simulink model "Ex9"  (R2019b)
settings: Solver=VariableStepAuto  StartTime=0.0  StopTime=0.003  RelTol=1e-3
values from neighbouring files (symbols this model uses):
  C = 1 / (L*Wn^2)    (= 2.29568411387e-06)    [Ex_27.m]    (also in Ex_29.m = 0.0001; Ex_5.m = 1e-06; Ex_8.m = 1e-05; Ex_9.m = 1e-05)
  L = 0.2    [Ex_23.m]    (also in Ex_27.m = 0.0001; Ex_29.m; Ex_8.m = 0.001; Ex_9.m = 0.001)
  R = 0.2    [Ex_21.m]    (also in Ex_22.m; Ex_23.m = 1.3; Ex_27.m = 2*qsi * sqrt(L/C); Ex_29.m = 1.3)
settings Model: Creator=andre  LastModifiedBy=andre

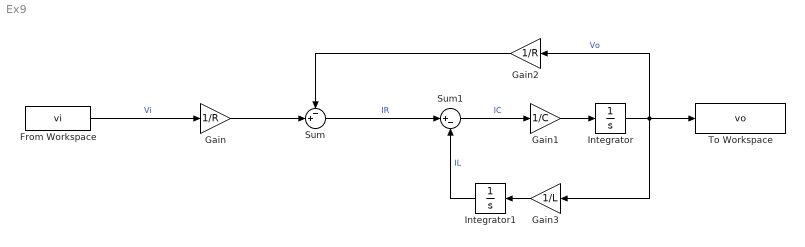
== system Ex9 ==
  From Workspace : FromWorkspace  VariableName=vi  SampleTime=0
  Gain : Gain  Gain=1/R
  Gain1 : Gain  Gain=1/C
  Gain2 : Gain  Gain=1/R
  Gain3 : Gain  Gain=1/L
  Integrator : Integrator
  Integrator1 : Integrator
  Sum : Sum  Inputs=-+|
  Sum1 : Sum  Inputs=|+-
  To Workspace : ToWorkspace  VariableName=vo  SaveFormat=Timeseries  SampleTime=-1
  wires:
  Sum1/1 -> Gain1/1  "IC"
  Gain1/1 -> Integrator/1
  Integrator/1 -> To Workspace/1, Gain3/1, Gain2/1  "Vo"
  Sum/1 -> Sum1/1  "IR"
  Gain/1 -> Sum/2
  Gain2/1 -> Sum/1
  Gain3/1 -> Integrator1/1
  Integrator1/1 -> Sum1/2  "IL"
  From Workspace/1 -> Gain/1  "Vi"
